simulink model "gravity"  (R2018b)
settings: Solver=VariableStepAuto  StartTime=0.0  StopTime=10.0  RelTol=1e-3
settings Model: Creator=Administrator  LastModifiedBy=Administrator

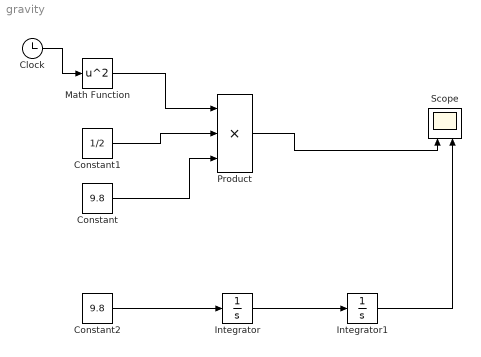
== system gravity ==
  Clock : Clock
  Constant : Constant  Value=9.8
  Constant1 : Constant  Value=1/2
  Constant2 : Constant  Value=9.8
  Integrator : Integrator  InitialCondition=-10
  Integrator1 : Integrator
  Math Function : Math  Operator=square  SaturateOnIntegerOverflow=on
  Product : Product  Inputs=3
  Scope : Scope  NumInputPorts=2
  wires:
  Clock/1 -> Math Function/1
  Math Function/1 -> Product/1
  Constant1/1 -> Product/2
  Constant/1 -> Product/3
  Product/1 -> Scope/1
  Constant2/1 -> Integrator/1
  Integrator/1 -> Integrator1/1
  Integrator1/1 -> Scope/2
